simulink model "Modelo_Discreto_SS_2914"  (R2014b)
settings: Solver=ode45  SolverMode=SingleTasking  StartTime=0.0  StopTime=10  RelTol=1e-3
undefined symbols (not defined in the file or in its folder): sigbuilder_block
libraries: simulink x1
settings Model: CovMetricSettings=dwe  CovHtmlReporting=off  covSaveCumulativeToWorkspaceVar=off  CovSaveSingleToWorkspaceVar=off  CovExternalEMLEnable=on  CovSFcnEnable=on  Creator=Steven  LastModifiedBy=PC-81597
settings DataIOCC: LimitDataPoints=off  SaveFormat=StructureWithTime
settings DebuggingCC: SolverPrmCheckMsg=none  FrameProcessingCompatibilityMsg=error  SFUnexpectedBacktrackingDiag=error  SFNoUnconditionalDefaultTransitionDiag=error
settings HardwareCC: ProdBitPerPointer=64  ProdLargestAtomicFloat=Float  ProdIntDivRoundTo=Zero  ProdEndianess=LittleEndian  ProdHWDeviceType=Specified
settings ModelReferenceCC: PropagateSignalLabelsOutOfModel=on
settings GRTTargetCC: TargetLangStandard=C99 (ISO)  GeneratePreprocessorConditionals=Use local settings

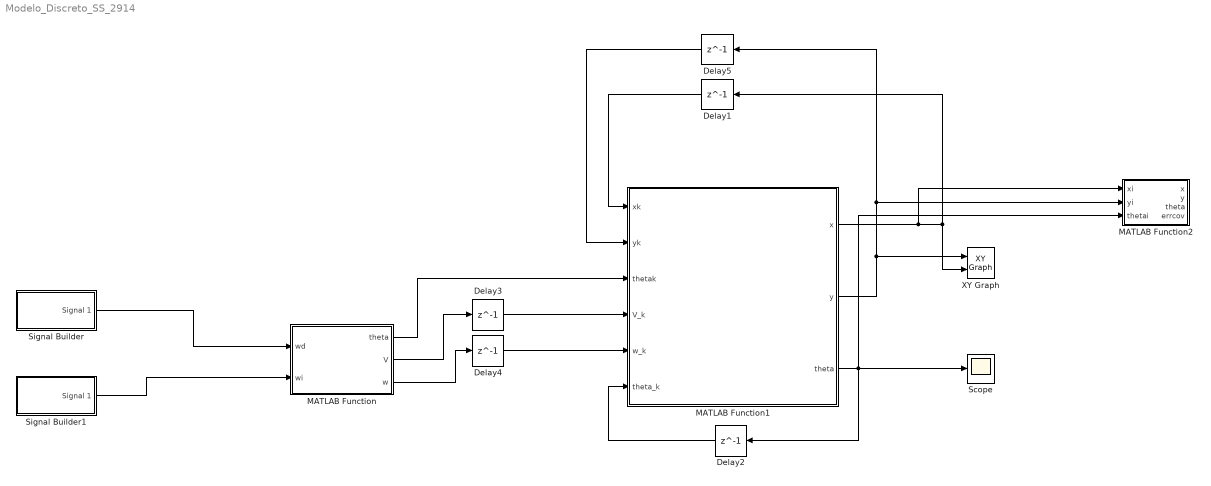
== system Modelo_Discreto_SS_2914 ==
  Delay{1..5} (5 alike) : Delay  DelayLength=1  InitialCondition=0  SampleTime=0.5
  MATLAB Function : MATLAB Function  TreatAsAtomicUnit=on
      settings: PermitHierarchicalResolution=ParametersOnly
  MATLAB Function1 : MATLAB Function  TreatAsAtomicUnit=on
      settings: PermitHierarchicalResolution=ParametersOnly
  MATLAB Function2 : MATLAB Function  TreatAsAtomicUnit=on
      settings: PermitHierarchicalResolution=ParametersOnly
  Scope : Scope
      settings: TimeRange=auto  MaxDataPoints=5000  SaveToWorkspace=off  SaveName=ScopeData  YMin=-1.00000  YMax=1.00000  SampleTime=-1
  Signal Builder : Subsystem  Tag=STV Subsys  LoadFcn=sigbuilder_block('load');  StartFcn=sigbuilder_block('start');  StopFcn=sigbuilder_block('stop');  ClipboardFcn=sigbuilder_block('clipboard');  mask(Sigbuilder block){}
      mask help: Simulink:masks:SigbuilderBlock_MD
      mask init:
      | if ~strcmp(get_param(bdroot(gcbh),'SimulationStatus'),'stopped') tuvar = sigbuilder_block('maskInit'); end
      settings: CopyFcn=sigbuilder_block('copy');  DeleteFcn=sigbuilder_block('delete');  ModelCloseFcn=sigbuilder_block('modelClose');  PreSaveFcn=sigbuilder_block('preSave');  PauseFcn=sigbuilder_block('pause');  ContinueFcn=sigbuilder_block('continue');  NameChangeFcn=sigbuilder_block('namechange');  OpenFcn=sigbuilder_block('open',[6 0 1012.5 453.75 ]);  CloseFcn=sigbuilder_block('close');
      mask Display: plot(0, 0, 100, 100,[2, 2, 32, 32, 2], [68, 8, 8, 68, 68],[32, 2], [38, 38], [32, 19, 2],[53, 60, 44], [32, 17, 17, 2],[16, 16, 31, 31]);txt = getActiveGroup(gcbh);text(2, 100, txt,'verticalAlignment', 'top');
  Signal Builder1 : Subsystem  Tag=STV Subsys  LoadFcn=sigbuilder_block('load');  StartFcn=sigbuilder_block('start');  StopFcn=sigbuilder_block('stop');  ClipboardFcn=sigbuilder_block('clipboard');  mask(Sigbuilder block){}
      mask help: Simulink:masks:SigbuilderBlock_MD
      mask init:
      | if ~strcmp(get_param(bdroot(gcbh),'SimulationStatus'),'stopped') tuvar = sigbuilder_block('maskInit'); end
      settings: CopyFcn=sigbuilder_block('copy');  DeleteFcn=sigbuilder_block('delete');  ModelCloseFcn=sigbuilder_block('modelClose');  PreSaveFcn=sigbuilder_block('preSave');  PauseFcn=sigbuilder_block('pause');  ContinueFcn=sigbuilder_block('continue');  NameChangeFcn=sigbuilder_block('namechange');  OpenFcn=sigbuilder_block('open',[0.75 0.75 510.75 487.5 ]);  CloseFcn=sigbuilder_block('close');
      mask Display: plot(0, 0, 100, 100,[2, 2, 32, 32, 2], [68, 8, 8, 68, 68],[32, 2], [38, 38], [32, 19, 2],[53, 60, 44], [32, 17, 17, 2],[16, 16, 31, 31]);txt = getActiveGroup(gcbh);text(2, 100, txt,'verticalAlignment', 'top');
  XY Graph : simulink/Sinks/XY Graph  xmin=-5  xmax=5  ymin=-10  ymax=10  st=0.5
  wires:
  Signal Builder/1(Signal 1) -> MATLAB Function/1(wd)
  Signal Builder1/1(Signal 1) -> MATLAB Function/2(wi)
  MATLAB Function/2(V) -> Delay3/1
  MATLAB Function/3(w) -> Delay4/1
  Delay4/1 -> MATLAB Function1/5(w_k)
  Delay3/1 -> MATLAB Function1/4(V_k)
  MATLAB Function1/3(theta) -> MATLAB Function2/3(thetai), Scope/1, Delay2/1
  Delay2/1 -> MATLAB Function1/6(theta_k)
  MATLAB Function/1(theta) -> MATLAB Function1/3(thetak)
  Delay1/1 -> MATLAB Function1/1(xk)
  MATLAB Function1/1(x) -> MATLAB Function2/1(xi), Delay1/1, XY Graph/2
  MATLAB Function1/2(y) -> MATLAB Function2/2(yi), Delay5/1, XY Graph/1
  Delay5/1 -> MATLAB Function1/2(yk)

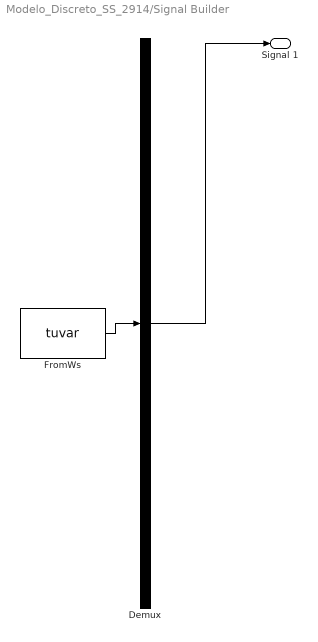
== system Modelo_Discreto_SS_2914/Signal Builder ==
  Demux : Demux  Tag=STV Demux  Outputs=1
  FromWs : FromWorkspace  Tag=STV FromWs  VariableName=tuvar  SampleTime=0
      SigBuilderData=|
      | common.afterFinalStr = 'Extrapolate'
      | common.sampleTime = 0
      | dataSet.timeRange = [0 100]
      | dataSet.name = 'Group 1'
      | sbobj.Groups.Name = 'Group 1'
      | sbobj.Groups.Signals.Name = 'Signal 1'
      | sbobj.Groups.Signals.XData = [0 100]
      | sbobj.Groups.Signals.YData = [0 9]
      | sbobj.Groups.TimeRange = [0 100]
  Signal 1 : Outport  Tag=STV Outport
  wires:
  Demux/1 -> Signal 1/1
  FromWs/1 -> Demux/1

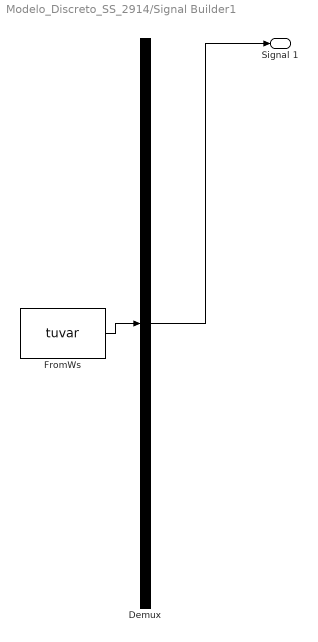
== system Modelo_Discreto_SS_2914/Signal Builder1 ==
  Demux : Demux  Tag=STV Demux  Outputs=1
  FromWs : FromWorkspace  Tag=STV FromWs  VariableName=tuvar  SampleTime=0
      SigBuilderData=|
      | common.afterFinalStr = 'Extrapolate'
      | common.sampleTime = 0
      | dataSet.timeRange = [0 100]
      | dataSet.name = 'Group 1'
      | sbobj.Groups.Name = 'Group 1'
      | sbobj.Groups.Signals.Name = 'Signal 1'
      | sbobj.Groups.Signals.XData = [0 100]
      | sbobj.Groups.Signals.YData = [0 9]
      | sbobj.Groups.TimeRange = [0 100]
  Signal 1 : Outport  Tag=STV Outport
  wires:
  Demux/1 -> Signal 1/1
  FromWs/1 -> Demux/1

== matlab function Modelo_Discreto_SS_2914/MATLAB Function1 ==
  data: x output; xk input; y output; yk input; thetak input; V_k input; w_k input; theta output; theta_k input
function [x,y,theta] = modelo_dis(xk,yk,thetak,V_k,w_k,theta_k)
Ts=0.5;
F=eye(3); %%matriz identidad
Fk= [xk;yk;thetak]; %% Las inicializamos en 0 ya que partimos desde el origen
B= [Ts*cos(theta_k) 0; Ts*sin(theta_k) 0; 0 Ts]; %%
u= [ V_k; w_k];

out = (F*Fk)+(B*u);
x=out(1);
y=out(2);
theta=out(3);

== matlab function Modelo_Discreto_SS_2914/MATLAB Function ==
  data: theta output; wd input; V output; wi input; w output
function [theta,V,w] = pre_proceso(wd,wi)
r=0.625;
b=19.5;
vi= r*wi;
vd= r*wd;
V = (vd+vi)/2;
w = (wi-wd)/b;
theta = w*r;

== matlab function Modelo_Discreto_SS_2914/MATLAB Function2 ==
  data: x output; xi input; y output; theta output; errcov output; yi input; thetai input
function [x,y,theta,errcov] = fcn(xi,yi,thetai)
%#codegen
Int = [xi yi thetai]
F=eye(3); 
H=eye(3);
persistent xe; % estados estimados, persistent para que lo mantenga en memoria
persistent P;
persistent K;
persistent R;
if isempty(xe)
        % R=diag(rand(3,1)); %aleatorio
        R=diag([225 16 0.04]); %del ejemplo
        xe = zeros(3,1);
end
if isempty(P)
        P=rand(3);
end

% esto debería ir en un ciclo infinito
% actualización en tiempo (predicción)
xe = F*xe;        % x[n+1|n]
P = F*P*F';     % P[n+1|n]

% actualización (medidas)
K = P*H'/(H*P*H'+R); % actualización de ganancia
xe = xe + K*(Int-H*xe);  % x[n|n]
P = (eye(3)-K.*H)*P;  % P[n|n]

ye=H*xe; %salida estimada
x=ye(1);
y=ye(2);
theta=ye(3);
errcov = H*P*H'; % actualización error covarianza
